simulink model "marine_otter_full"  (R2024a)
settings: Solver=FixedStepAuto  StartTime=0.0  StopTime=10.0  FixedStep=0.05  RelTol=1e-3
PostLoadFcn:
  | on_model_load
InitFcn:
  | on_model_start
StopFcn:
  | on_simulation_done
undefined symbols (not defined in the file or in its folder): ActiveExperiment
libraries: marine_lib_sys x5, data_driven_lib_ctl x3, csbenchlab_ctl x2
PostSaveFcn:
  | on_model_save
settings Model: Creator=luka  LastModifiedBy=luka

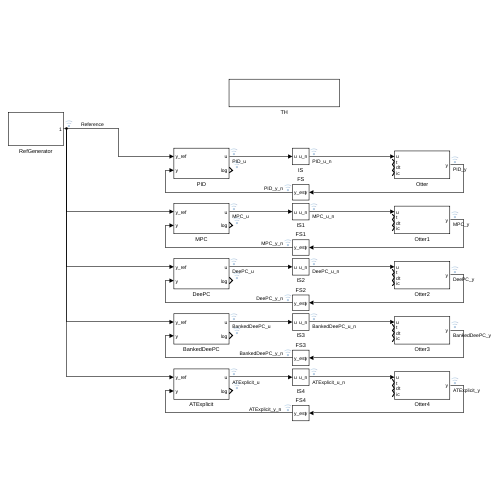
[thumbnail: Simulink's stored preview of the top-level diagram]
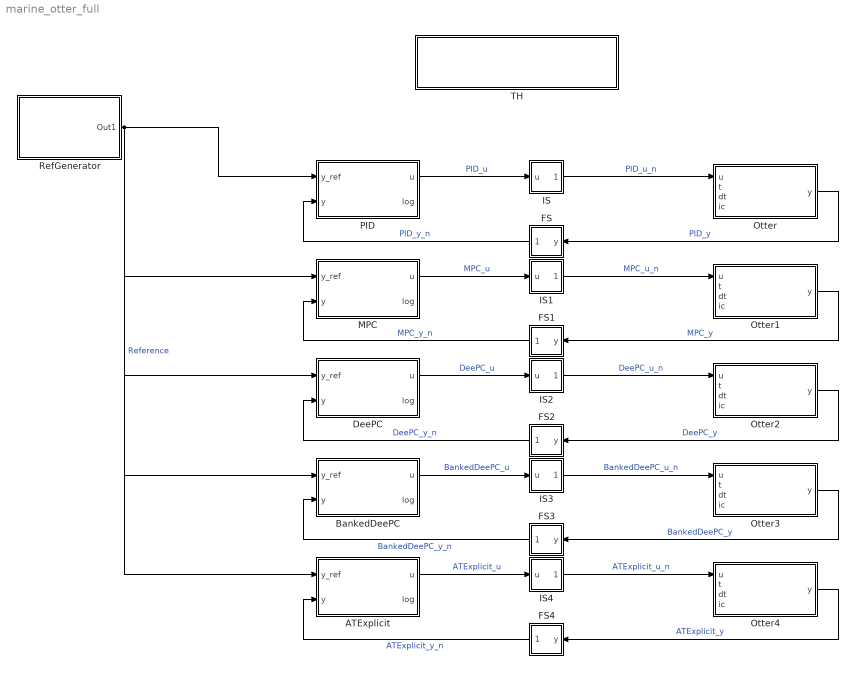
== system marine_otter_full ==
  ATExplicit : Subsystem  Tag=__cs_template;__cs_comptype:ctl
      mask DialogControl ParameterGroupVar Prompt: Params
  BankedDeePC : Subsystem  Tag=__cs_template;__cs_comptype:ctl
      mask DialogControl ParameterGroupVar Prompt: Params
  DeePC : Subsystem  Tag=__cs_template;__cs_comptype:ctl
      mask DialogControl ParameterGroupVar Prompt: Params
  FS : Subsystem
  FS1 : Subsystem
  FS2 : Subsystem
  FS3 : Subsystem
  FS4 : Subsystem
  IS : Subsystem
  IS1 : Subsystem
  IS2 : Subsystem
  IS3 : Subsystem
  IS4 : Subsystem
  MPC : Subsystem  Tag=__cs_template;__cs_comptype:ctl
      mask DialogControl ParameterGroupVar Prompt: Params
  Otter : Subsystem  Tag=__cs_template;__cs_comptype:sys
      mask DialogControl ParameterGroupVar Prompt: Params
  Otter1 : Subsystem  Tag=__cs_template;__cs_comptype:sys
      mask DialogControl ParameterGroupVar Prompt: Params
  Otter2 : Subsystem  Tag=__cs_template;__cs_comptype:sys
      mask DialogControl ParameterGroupVar Prompt: Params
  Otter3 : Subsystem  Tag=__cs_template;__cs_comptype:sys
      mask DialogControl ParameterGroupVar Prompt: Params
  Otter4 : Subsystem  Tag=__cs_template;__cs_comptype:sys
      mask DialogControl ParameterGroupVar Prompt: Params
  PID : Subsystem  Tag=__cs_template;__cs_comptype:ctl
      mask DialogControl ParameterGroupVar Prompt: Params
  RefGenerator : Subsystem  mask{experiment=P1}
      settings: OpenFcn=on_reference_generator_open();
      mask TypeOptions experiment: P1
      mask Callback experiment: on_experiment_select;
      mask DialogControl DescGroupVar Prompt: Select experiment
  TH : Subsystem
      mask DialogControl ParameterGroupVar Prompt: Params
  wires:
  PID/1(u) -> IS/1(u)  "PID_u"
  IS/1(u_n) -> Otter/1(u)  "PID_u_n"
  Otter/1(y) -> FS/1(y)  "PID_y"
  FS/1(y_est) -> PID/2(y)  "PID_y_n"
  RefGenerator/1(Out1) -> PID/1(y_ref), MPC/1(y_ref), DeePC/1(y_ref), BankedDeePC/1(y_ref), ATExplicit/1(y_ref)  "Reference"
  MPC/1(u) -> IS1/1(u)  "MPC_u"
  IS1/1(u_n) -> Otter1/1(u)  "MPC_u_n"
  Otter1/1(y) -> FS1/1(y)  "MPC_y"
  FS1/1(y_est) -> MPC/2(y)  "MPC_y_n"
  DeePC/1(u) -> IS2/1(u)  "DeePC_u"
  IS2/1(u_n) -> Otter2/1(u)  "DeePC_u_n"
  Otter2/1(y) -> FS2/1(y)  "DeePC_y"
  FS2/1(y_est) -> DeePC/2(y)  "DeePC_y_n"
  BankedDeePC/1(u) -> IS3/1(u)  "BankedDeePC_u"
  IS3/1(u_n) -> Otter3/1(u)  "BankedDeePC_u_n"
  Otter3/1(y) -> FS3/1(y)  "BankedDeePC_y"
  FS3/1(y_est) -> BankedDeePC/2(y)  "BankedDeePC_y_n"
  ATExplicit/1(u) -> IS4/1(u)  "ATExplicit_u"
  IS4/1(u_n) -> Otter4/1(u)  "ATExplicit_u_n"
  Otter4/1(y) -> FS4/1(y)  "ATExplicit_y"
  FS4/1(y_est) -> ATExplicit/2(y)  "ATExplicit_y_n"

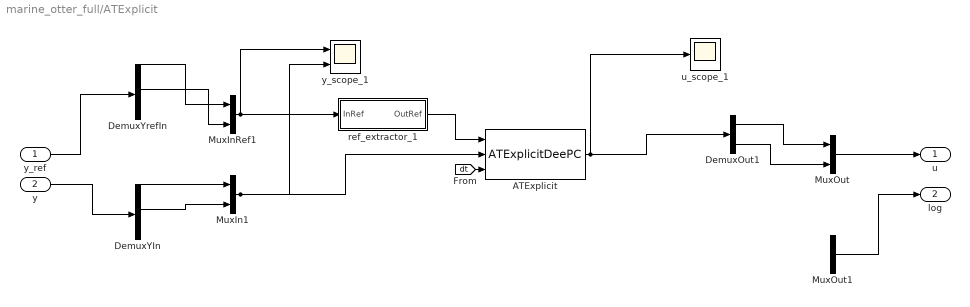
== system marine_otter_full/ATExplicit ==
  y_ref : Inport  PortDimensions=12
  y : Inport  Port=2  PortDimensions=12
  ATExplicit : data_driven_lib_ctl/ATExplicitDeePC  Tag=__cs_comptype:ctl;__cs_compimpl:mat;  iid__=[51 50 99 48 56 97 99 98 45 57 52 54 52 45 52 97 98 97 45 97 97 97 101 45 49 100 57 57 102 51 57 52 98 51 53 48]  pid__=[65 84 69 120 112 108 105 99 105 116 68 101 101 80 67 58 100 97 116 97 95 100 114 105 118 101 110 95 108 105 98]  params=marine_otter_full_params.ctl.ATExplicit  data=ATExplicitDeePC_data  ParamsType=ATExplicitDeePC_PT  DataType=ATExplicitDeePC_DT  u_ic=0
  DemuxOut1 : Demux  Outputs=2
  DemuxYIn : Demux  Outputs=12
  DemuxYrefIn : Demux  Outputs=12
  MuxIn1 : Mux  Inputs=2
  MuxInRef1 : Mux  Inputs=2
  MuxOut : Mux  Inputs=2
  MuxOut1 : BusCreator  Inputs=1
  ref_extractor_1 : Subsystem
  u_scope_1 : Scope
  y_scope_1 : Scope  NumInputPorts=2
  u : Outport  PortDimensions=2
  log : Outport  Port=2
  wires:
  [dt] -> ATExplicit/3
  y/1 -> DemuxYIn/1
  y_ref/1 -> DemuxYrefIn/1
  MuxOut/1 -> u/1
  MuxOut1/1 -> log/1
  MuxInRef1/1 -> ref_extractor_1/1(InRef), y_scope_1/1
  ref_extractor_1/1(OutRef) -> ATExplicit/1
  MuxIn1/1 -> ATExplicit/2, y_scope_1/2
  ATExplicit/1 -> DemuxOut1/1, u_scope_1/1
  DemuxYIn/1 -> MuxIn1/1
  DemuxYrefIn/1 -> MuxInRef1/1
  DemuxYIn/6 -> MuxIn1/2
  DemuxYrefIn/6 -> MuxInRef1/2
  DemuxOut1/1 -> MuxOut/1
  DemuxOut1/2 -> MuxOut/2

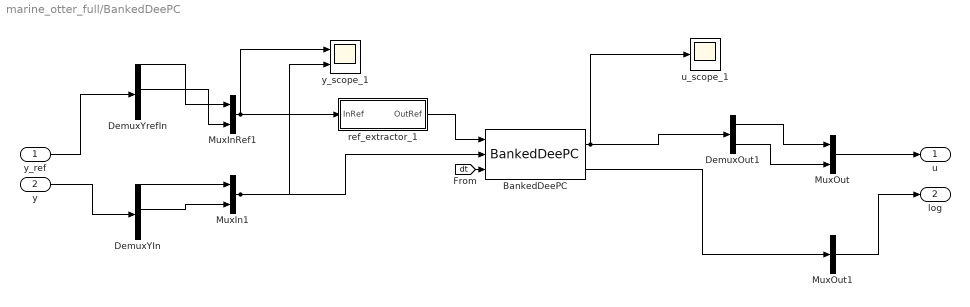
== system marine_otter_full/BankedDeePC ==
  y_ref : Inport  PortDimensions=12
  y : Inport  Port=2  PortDimensions=12
  BankedDeePC : data_driven_lib_ctl/BankedDeePC  Tag=__cs_comptype:ctl;__cs_compimpl:mat;  iid__=[54 56 49 56 55 102 55 100 45 56 49 102 53 45 52 55 53 54 45 57 54 98 101 45 100 101 48 100 54 53 51 54 51 97 54 51]  pid__=[66 97 110 107 101 100 68 101 101 80 67 58 100 97 116 97 95 100 114 105 118 101 110 95 108 105 98]  params=marine_otter_full_params.ctl.BankedDeePC  LogEntryType=BankedDeePC_LT  data=BankedDeePC_data  ParamsType=BankedDeePC_PT  DataType=BankedDeePC_DT  u_ic=0
  DemuxOut1 : Demux  Outputs=2
  DemuxYIn : Demux  Outputs=12
  DemuxYrefIn : Demux  Outputs=12
  MuxIn1 : Mux  Inputs=2
  MuxInRef1 : Mux  Inputs=2
  MuxOut : Mux  Inputs=2
  MuxOut1 : BusCreator  Inputs=1
  ref_extractor_1 : Subsystem
  u_scope_1 : Scope
  y_scope_1 : Scope  NumInputPorts=2
  u : Outport  PortDimensions=2
  log : Outport  Port=2
  wires:
  [dt] -> BankedDeePC/3
  y/1 -> DemuxYIn/1
  y_ref/1 -> DemuxYrefIn/1
  MuxOut/1 -> u/1
  MuxOut1/1 -> log/1
  MuxInRef1/1 -> ref_extractor_1/1(InRef), y_scope_1/1
  ref_extractor_1/1(OutRef) -> BankedDeePC/1
  MuxIn1/1 -> BankedDeePC/2, y_scope_1/2
  BankedDeePC/1 -> DemuxOut1/1, u_scope_1/1
  BankedDeePC/2 -> MuxOut1/1
  DemuxYIn/1 -> MuxIn1/1
  DemuxYrefIn/1 -> MuxInRef1/1
  DemuxYIn/6 -> MuxIn1/2
  DemuxYrefIn/6 -> MuxInRef1/2
  DemuxOut1/1 -> MuxOut/1
  DemuxOut1/2 -> MuxOut/2

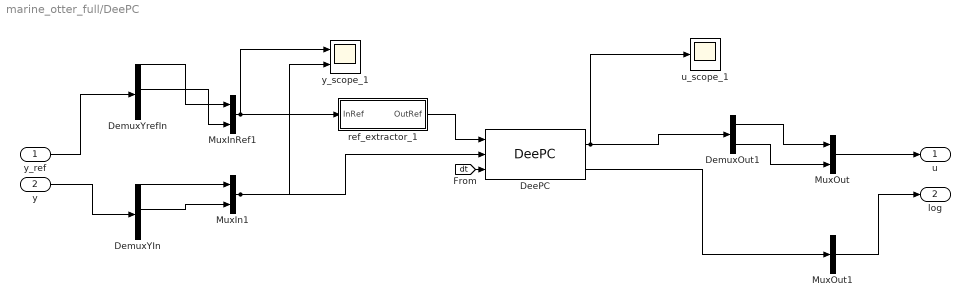
== system marine_otter_full/DeePC ==
  y_ref : Inport  PortDimensions=12
  y : Inport  Port=2  PortDimensions=12
  DeePC : data_driven_lib_ctl/DeePC  Tag=__cs_comptype:ctl;__cs_compimpl:mat;  iid__=[102 52 49 101 102 57 101 52 45 98 97 51 52 45 52 49 54 99 45 56 52 98 54 45 55 55 57 52 57 53 54 97 51 99 48 52]  pid__=[68 101 101 80 67 58 100 97 116 97 95 100 114 105 118 101 110 95 108 105 98]  params=marine_otter_full_params.ctl.DeePC  LogEntryType=DeePC_LT  data=DeePC_data  ParamsType=DeePC_PT  DataType=DeePC_DT  u_ic=0
  DemuxOut1 : Demux  Outputs=2
  DemuxYIn : Demux  Outputs=12
  DemuxYrefIn : Demux  Outputs=12
  MuxIn1 : Mux  Inputs=2
  MuxInRef1 : Mux  Inputs=2
  MuxOut : Mux  Inputs=2
  MuxOut1 : BusCreator  Inputs=1
  ref_extractor_1 : Subsystem
  u_scope_1 : Scope
  y_scope_1 : Scope  NumInputPorts=2
  u : Outport  PortDimensions=2
  log : Outport  Port=2
  wires:
  [dt] -> DeePC/3
  y/1 -> DemuxYIn/1
  y_ref/1 -> DemuxYrefIn/1
  MuxOut/1 -> u/1
  MuxOut1/1 -> log/1
  MuxInRef1/1 -> ref_extractor_1/1(InRef), y_scope_1/1
  ref_extractor_1/1(OutRef) -> DeePC/1
  MuxIn1/1 -> DeePC/2, y_scope_1/2
  DeePC/1 -> DemuxOut1/1, u_scope_1/1
  DeePC/2 -> MuxOut1/1
  DemuxYIn/1 -> MuxIn1/1
  DemuxYrefIn/1 -> MuxInRef1/1
  DemuxYIn/6 -> MuxIn1/2
  DemuxYrefIn/6 -> MuxInRef1/2
  DemuxOut1/1 -> MuxOut/1
  DemuxOut1/2 -> MuxOut/2

== system marine_otter_full/FS ==
  y : Inport
  CS Dist : Subsystem
      mask DialogControl ParameterGroupVar Prompt: Params
  CS Est : Subsystem
      mask DialogControl ParameterGroupVar Prompt: Params
  y_est : Outport
  wires:
  CS Est/1(y_est) -> y_est/1
  CS Dist/1(y_n) -> CS Est/1(y)
  y/1 -> CS Dist/1(y)

== system marine_otter_full/FS1 ==
  y : Inport
  CS Dist : Subsystem
      mask DialogControl ParameterGroupVar Prompt: Params
  CS Est : Subsystem
      mask DialogControl ParameterGroupVar Prompt: Params
  y_est : Outport
  wires:
  CS Est/1(y_est) -> y_est/1
  CS Dist/1(y_n) -> CS Est/1(y)
  y/1 -> CS Dist/1(y)

== system marine_otter_full/FS2 ==
  y : Inport
  CS Dist : Subsystem
      mask DialogControl ParameterGroupVar Prompt: Params
  CS Est : Subsystem
      mask DialogControl ParameterGroupVar Prompt: Params
  y_est : Outport
  wires:
  CS Est/1(y_est) -> y_est/1
  CS Dist/1(y_n) -> CS Est/1(y)
  y/1 -> CS Dist/1(y)

== system marine_otter_full/FS3 ==
  y : Inport
  CS Dist : Subsystem
      mask DialogControl ParameterGroupVar Prompt: Params
  CS Est : Subsystem
      mask DialogControl ParameterGroupVar Prompt: Params
  y_est : Outport
  wires:
  CS Est/1(y_est) -> y_est/1
  CS Dist/1(y_n) -> CS Est/1(y)
  y/1 -> CS Dist/1(y)

== system marine_otter_full/FS4 ==
  y : Inport
  CS Dist : Subsystem
      mask DialogControl ParameterGroupVar Prompt: Params
  CS Est : Subsystem
      mask DialogControl ParameterGroupVar Prompt: Params
  y_est : Outport
  wires:
  CS Est/1(y_est) -> y_est/1
  CS Dist/1(y_n) -> CS Est/1(y)
  y/1 -> CS Dist/1(y)

== system marine_otter_full/IS ==
  u : Inport
  CS Dist : Subsystem
      mask DialogControl ParameterGroupVar Prompt: Params
  u_n : Outport
  wires:
  CS Dist/1(y_n) -> u_n/1
  u/1 -> CS Dist/1(y)

== system marine_otter_full/IS1 ==
  u : Inport
  CS Dist : Subsystem
      mask DialogControl ParameterGroupVar Prompt: Params
  u_n : Outport
  wires:
  CS Dist/1(y_n) -> u_n/1
  u/1 -> CS Dist/1(y)

== system marine_otter_full/IS2 ==
  u : Inport
  CS Dist : Subsystem
      mask DialogControl ParameterGroupVar Prompt: Params
  u_n : Outport
  wires:
  CS Dist/1(y_n) -> u_n/1
  u/1 -> CS Dist/1(y)

== system marine_otter_full/IS3 ==
  u : Inport
  CS Dist : Subsystem
      mask DialogControl ParameterGroupVar Prompt: Params
  u_n : Outport
  wires:
  CS Dist/1(y_n) -> u_n/1
  u/1 -> CS Dist/1(y)

== system marine_otter_full/IS4 ==
  u : Inport
  CS Dist : Subsystem
      mask DialogControl ParameterGroupVar Prompt: Params
  u_n : Outport
  wires:
  CS Dist/1(y_n) -> u_n/1
  u/1 -> CS Dist/1(y)

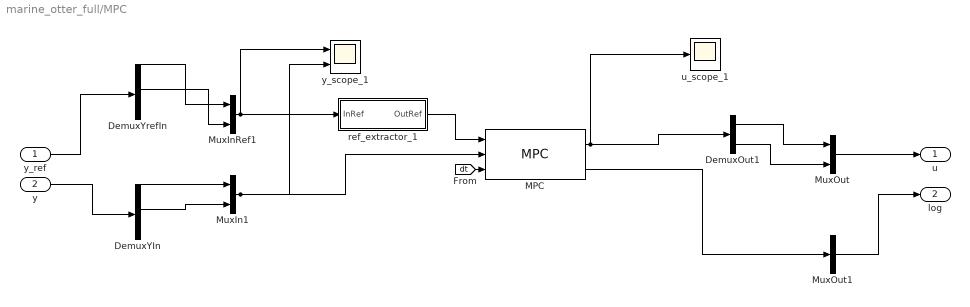
== system marine_otter_full/MPC ==
  y_ref : Inport  PortDimensions=12
  y : Inport  Port=2  PortDimensions=12
  DemuxOut1 : Demux  Outputs=2
  DemuxYIn : Demux  Outputs=12
  DemuxYrefIn : Demux  Outputs=12
  MPC : csbenchlab_ctl/MPC  Tag=__cs_slx_ctl;__cs_comptype:ctl;__cs_compimpl:slx;  mpc_path=0  out_gain=0  iid__=[56 49 102 99 48 101 54 102 45 50 51 56 52 45 52 57 54 57 45 97 98 51 51 45 52 99 99 48 98 52 97 56 56 100 97 99]  pid__=[77 80 67 58 99 115 98 101 110 99 104 108 97 98]  params=marine_otter_full_params.ctl.MPC  params_struct_name=marine_otter_full_params.ctl.MPC
  MuxIn1 : Mux  Inputs=2
  MuxInRef1 : Mux  Inputs=2
  MuxOut : Mux  Inputs=2
  MuxOut1 : BusCreator  Inputs=1
  ref_extractor_1 : Subsystem
  u_scope_1 : Scope
  y_scope_1 : Scope  NumInputPorts=2
  u : Outport  PortDimensions=2
  log : Outport  Port=2
  wires:
  [dt] -> MPC/3
  y/1 -> DemuxYIn/1
  y_ref/1 -> DemuxYrefIn/1
  MuxOut/1 -> u/1
  MuxOut1/1 -> log/1
  MuxInRef1/1 -> ref_extractor_1/1(InRef), y_scope_1/1
  ref_extractor_1/1(OutRef) -> MPC/1
  MuxIn1/1 -> MPC/2, y_scope_1/2
  MPC/1 -> DemuxOut1/1, u_scope_1/1
  MPC/2 -> MuxOut1/1
  DemuxYIn/1 -> MuxIn1/1
  DemuxYrefIn/1 -> MuxInRef1/1
  DemuxYIn/6 -> MuxIn1/2
  DemuxYrefIn/6 -> MuxInRef1/2
  DemuxOut1/1 -> MuxOut/1
  DemuxOut1/2 -> MuxOut/2

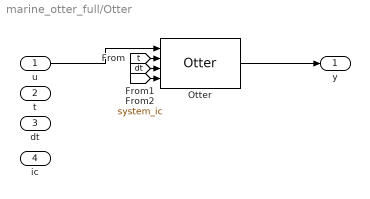
== system marine_otter_full/Otter ==
  u : Inport
  t : Inport  Port=2
  dt : Inport  Port=3
  ic : Inport  Port=4
  Otter : marine_lib_sys/Otter  Tag=system;__cs_slx_sys;__cs_comptype:sys;__cs_compimpl:slx;  payload_mass=0  payload_location=[0,0, 0]  current_speed=0  current_direction=0  out_gain=1  iid__=[52 97 48 100 49 48 49 48 45 52 53 52 57 45 52 100 53 49 45 98 51 97 53 45 54 48 50 101 55 99 57 51 50 98 52 53]  pid__=[79 116 116 101 114 58 109 97 114 105 110 101 95 108 105 98]  params=ActiveExperiment.SystemParams  params_struct_name=marine_otter_full_params.sys.Otter
  y : Outport
  wires:
  u/1 -> Otter/1
  Otter/1 -> y/1
  [t] -> Otter/2
  [dt] -> Otter/3
  [system_ic] -> Otter/4

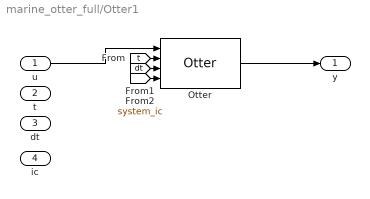
== system marine_otter_full/Otter1 ==
  u : Inport
  t : Inport  Port=2
  dt : Inport  Port=3
  ic : Inport  Port=4
  Otter : marine_lib_sys/Otter  Tag=system;__cs_slx_sys;__cs_comptype:sys;__cs_compimpl:slx;  payload_mass=0  payload_location=[0,0, 0]  current_speed=0  current_direction=0  out_gain=1  iid__=[52 97 48 100 49 48 49 48 45 52 53 52 57 45 52 100 53 49 45 98 51 97 53 45 54 48 50 101 55 99 57 51 50 98 52 53]  pid__=[79 116 116 101 114 58 109 97 114 105 110 101 95 108 105 98]  params=ActiveExperiment.SystemParams  params_struct_name=marine_otter_full_params.sys.Otter
  y : Outport
  wires:
  u/1 -> Otter/1
  Otter/1 -> y/1
  [t] -> Otter/2
  [dt] -> Otter/3
  [system_ic] -> Otter/4

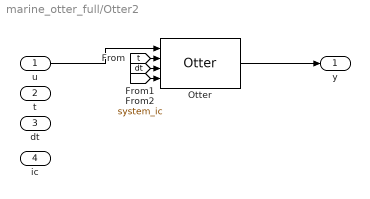
== system marine_otter_full/Otter2 ==
  u : Inport
  t : Inport  Port=2
  dt : Inport  Port=3
  ic : Inport  Port=4
  Otter : marine_lib_sys/Otter  Tag=system;__cs_slx_sys;__cs_comptype:sys;__cs_compimpl:slx;  payload_mass=0  payload_location=[0,0, 0]  current_speed=0  current_direction=0  out_gain=1  iid__=[52 97 48 100 49 48 49 48 45 52 53 52 57 45 52 100 53 49 45 98 51 97 53 45 54 48 50 101 55 99 57 51 50 98 52 53]  pid__=[79 116 116 101 114 58 109 97 114 105 110 101 95 108 105 98]  params=ActiveExperiment.SystemParams  params_struct_name=marine_otter_full_params.sys.Otter
  y : Outport
  wires:
  u/1 -> Otter/1
  Otter/1 -> y/1
  [t] -> Otter/2
  [dt] -> Otter/3
  [system_ic] -> Otter/4

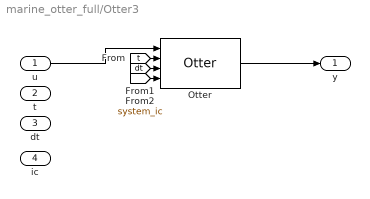
== system marine_otter_full/Otter3 ==
  u : Inport
  t : Inport  Port=2
  dt : Inport  Port=3
  ic : Inport  Port=4
  Otter : marine_lib_sys/Otter  Tag=system;__cs_slx_sys;__cs_comptype:sys;__cs_compimpl:slx;  payload_mass=0  payload_location=[0,0, 0]  current_speed=0  current_direction=0  out_gain=1  iid__=[52 97 48 100 49 48 49 48 45 52 53 52 57 45 52 100 53 49 45 98 51 97 53 45 54 48 50 101 55 99 57 51 50 98 52 53]  pid__=[79 116 116 101 114 58 109 97 114 105 110 101 95 108 105 98]  params=ActiveExperiment.SystemParams  params_struct_name=marine_otter_full_params.sys.Otter
  y : Outport
  wires:
  u/1 -> Otter/1
  Otter/1 -> y/1
  [t] -> Otter/2
  [dt] -> Otter/3
  [system_ic] -> Otter/4

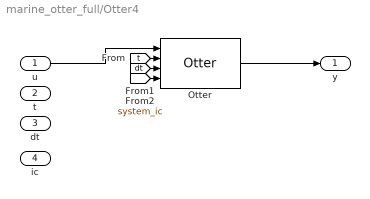
== system marine_otter_full/Otter4 ==
  u : Inport
  t : Inport  Port=2
  dt : Inport  Port=3
  ic : Inport  Port=4
  Otter : marine_lib_sys/Otter  Tag=system;__cs_slx_sys;__cs_comptype:sys;__cs_compimpl:slx;  payload_mass=0  payload_location=[0,0, 0]  current_speed=0  current_direction=0  out_gain=1  iid__=[52 97 48 100 49 48 49 48 45 52 53 52 57 45 52 100 53 49 45 98 51 97 53 45 54 48 50 101 55 99 57 51 50 98 52 53]  pid__=[79 116 116 101 114 58 109 97 114 105 110 101 95 108 105 98]  params=ActiveExperiment.SystemParams  params_struct_name=marine_otter_full_params.sys.Otter
  y : Outport
  wires:
  u/1 -> Otter/1
  Otter/1 -> y/1
  [t] -> Otter/2
  [dt] -> Otter/3
  [system_ic] -> Otter/4

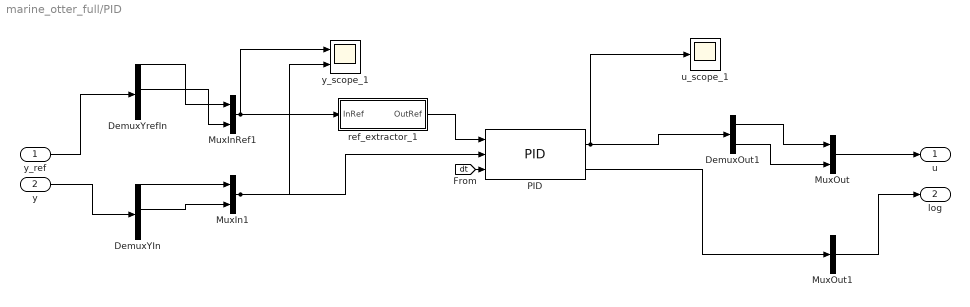
== system marine_otter_full/PID ==
  y_ref : Inport  PortDimensions=12
  y : Inport  Port=2  PortDimensions=12
  DemuxOut1 : Demux  Outputs=2
  DemuxYIn : Demux  Outputs=12
  DemuxYrefIn : Demux  Outputs=12
  MuxIn1 : Mux  Inputs=2
  MuxInRef1 : Mux  Inputs=2
  MuxOut : Mux  Inputs=2
  MuxOut1 : BusCreator  Inputs=1
  PID : csbenchlab_ctl/PID  Tag=__cs_slx_ctl;__cs_comptype:ctl;__cs_compimpl:slx;  K_p=K_p  K_i=K_i  K_d=K_d  K_N=K_N  saturation_min=saturation_min  saturation_max=saturation_max  iid__=[56 53 56 50 101 51 101 49 45 100 101 56 53 45 52 54 54 101 45 98 52 49 50 45 52 52 97 50 54 57 99 99 100 50 98 102]  pid__=[80 73 68 58 99 115 98 101 110 99 104 108 97 98]  params=marine_otter_full_params.ctl.PID  params_struct_name=marine_otter_full_params.ctl.PID
  ref_extractor_1 : Subsystem
  u_scope_1 : Scope
  y_scope_1 : Scope  NumInputPorts=2
  u : Outport  PortDimensions=2
  log : Outport  Port=2
  wires:
  [dt] -> PID/3
  y/1 -> DemuxYIn/1
  y_ref/1 -> DemuxYrefIn/1
  MuxOut/1 -> u/1
  MuxOut1/1 -> log/1
  MuxInRef1/1 -> ref_extractor_1/1(InRef), y_scope_1/1
  ref_extractor_1/1(OutRef) -> PID/1
  MuxIn1/1 -> PID/2, y_scope_1/2
  PID/1 -> DemuxOut1/1, u_scope_1/1
  PID/2 -> MuxOut1/1
  DemuxYIn/1 -> MuxIn1/1
  DemuxYrefIn/1 -> MuxInRef1/1
  DemuxYIn/6 -> MuxIn1/2
  DemuxYrefIn/6 -> MuxInRef1/2
  DemuxOut1/1 -> MuxOut/1
  DemuxOut1/2 -> MuxOut/2

== system marine_otter_full/RefGenerator ==
  IC : Constant  Value=ActiveExperiment.SystemIc
  ReferenceFile : FromFile  SampleTime=0
  Out1 : Outport
  tag scope: system_ic=global
  wires:
  IC/1 -> [system_ic]
  ReferenceFile/1 -> Out1/1

== system marine_otter_full/TH ==
  Clock : Clock
  Constant : Constant
  Memory : Memory
  Subtract : Sum  Inputs=+-
  tag scope: dt=global, t=global
  wires:
  Subtract/1 -> [dt]
  Memory/1 -> Subtract/2
  Clock/1 -> Memory/1, Subtract/1, [t]

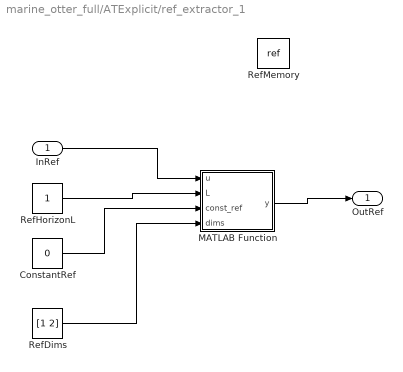
== system marine_otter_full/ATExplicit/ref_extractor_1 ==
  InRef : Inport
  ConstantRef : Constant  Value=0
  MATLAB Function : MATLAB Function  TreatAsAtomicUnit=on
  RefDims : Constant  Value=[1 2]
  RefHorizonL : Constant
  RefMemory : DataStoreMemory  DataStoreName=ref  WriteAfterWriteMsg=warning  ShowAdditionalParam=off  OutDataTypeStr=double
  OutRef : Outport
  wires:
  ConstantRef/1 -> MATLAB Function/3(const_ref)
  RefDims/1 -> MATLAB Function/4(dims)
  RefHorizonL/1 -> MATLAB Function/2(L)
  InRef/1 -> MATLAB Function/1(u)
  MATLAB Function/1(y) -> OutRef/1

== system marine_otter_full/BankedDeePC/ref_extractor_1 ==
  InRef : Inport
  ConstantRef : Constant  Value=0
  MATLAB Function : MATLAB Function  TreatAsAtomicUnit=on
  RefDims : Constant  Value=[1 2]
  RefHorizonL : Constant
  RefMemory : DataStoreMemory  DataStoreName=ref  WriteAfterWriteMsg=warning  ShowAdditionalParam=off  OutDataTypeStr=double
  OutRef : Outport
  wires:
  ConstantRef/1 -> MATLAB Function/3(const_ref)
  RefDims/1 -> MATLAB Function/4(dims)
  RefHorizonL/1 -> MATLAB Function/2(L)
  InRef/1 -> MATLAB Function/1(u)
  MATLAB Function/1(y) -> OutRef/1

== system marine_otter_full/DeePC/ref_extractor_1 ==
  InRef : Inport
  ConstantRef : Constant  Value=0
  MATLAB Function : MATLAB Function  TreatAsAtomicUnit=on
  RefDims : Constant  Value=[1 2]
  RefHorizonL : Constant
  RefMemory : DataStoreMemory  DataStoreName=ref  WriteAfterWriteMsg=warning  ShowAdditionalParam=off  OutDataTypeStr=double
  OutRef : Outport
  wires:
  ConstantRef/1 -> MATLAB Function/3(const_ref)
  RefDims/1 -> MATLAB Function/4(dims)
  RefHorizonL/1 -> MATLAB Function/2(L)
  InRef/1 -> MATLAB Function/1(u)
  MATLAB Function/1(y) -> OutRef/1

== system marine_otter_full/FS/CS Dist ==
  y : Inport
  Gain : Gain
  y_n : Outport
  wires:
  Gain/1 -> y_n/1
  y/1 -> Gain/1

== system marine_otter_full/FS/CS Est ==
  y : Inport
  Gain : Gain
  y_est : Outport
  wires:
  y/1 -> Gain/1
  Gain/1 -> y_est/1

== system marine_otter_full/FS1/CS Dist ==
  y : Inport
  Gain : Gain
  y_n : Outport
  wires:
  Gain/1 -> y_n/1
  y/1 -> Gain/1

== system marine_otter_full/FS1/CS Est ==
  y : Inport
  Gain : Gain
  y_est : Outport
  wires:
  y/1 -> Gain/1
  Gain/1 -> y_est/1

== system marine_otter_full/FS2/CS Dist ==
  y : Inport
  Gain : Gain
  y_n : Outport
  wires:
  Gain/1 -> y_n/1
  y/1 -> Gain/1

== system marine_otter_full/FS2/CS Est ==
  y : Inport
  Gain : Gain
  y_est : Outport
  wires:
  y/1 -> Gain/1
  Gain/1 -> y_est/1

== system marine_otter_full/FS3/CS Dist ==
  y : Inport
  Gain : Gain
  y_n : Outport
  wires:
  Gain/1 -> y_n/1
  y/1 -> Gain/1

== system marine_otter_full/FS3/CS Est ==
  y : Inport
  Gain : Gain
  y_est : Outport
  wires:
  y/1 -> Gain/1
  Gain/1 -> y_est/1

== system marine_otter_full/FS4/CS Dist ==
  y : Inport
  Gain : Gain
  y_n : Outport
  wires:
  Gain/1 -> y_n/1
  y/1 -> Gain/1

== system marine_otter_full/FS4/CS Est ==
  y : Inport
  Gain : Gain
  y_est : Outport
  wires:
  y/1 -> Gain/1
  Gain/1 -> y_est/1

== system marine_otter_full/IS/CS Dist ==
  y : Inport
  Gain : Gain
  y_n : Outport
  wires:
  y/1 -> Gain/1
  Gain/1 -> y_n/1

== system marine_otter_full/IS1/CS Dist ==
  y : Inport
  Gain : Gain
  y_n : Outport
  wires:
  y/1 -> Gain/1
  Gain/1 -> y_n/1

== system marine_otter_full/IS2/CS Dist ==
  y : Inport
  Gain : Gain
  y_n : Outport
  wires:
  y/1 -> Gain/1
  Gain/1 -> y_n/1

== system marine_otter_full/IS3/CS Dist ==
  y : Inport
  Gain : Gain
  y_n : Outport
  wires:
  y/1 -> Gain/1
  Gain/1 -> y_n/1

== system marine_otter_full/IS4/CS Dist ==
  y : Inport
  Gain : Gain
  y_n : Outport
  wires:
  y/1 -> Gain/1
  Gain/1 -> y_n/1

== system marine_otter_full/MPC/ref_extractor_1 ==
  InRef : Inport
  ConstantRef : Constant  Value=0
  MATLAB Function : MATLAB Function  TreatAsAtomicUnit=on
  RefDims : Constant  Value=[1 2]
  RefHorizonL : Constant
  RefMemory : DataStoreMemory  DataStoreName=ref  WriteAfterWriteMsg=warning  ShowAdditionalParam=off  OutDataTypeStr=double
  OutRef : Outport
  wires:
  ConstantRef/1 -> MATLAB Function/3(const_ref)
  RefDims/1 -> MATLAB Function/4(dims)
  RefHorizonL/1 -> MATLAB Function/2(L)
  InRef/1 -> MATLAB Function/1(u)
  MATLAB Function/1(y) -> OutRef/1

== system marine_otter_full/PID/ref_extractor_1 ==
  InRef : Inport
  ConstantRef : Constant  Value=0
  MATLAB Function : MATLAB Function  TreatAsAtomicUnit=on
  RefDims : Constant  Value=[1 2]
  RefHorizonL : Constant
  RefMemory : DataStoreMemory  DataStoreName=ref  WriteAfterWriteMsg=warning  ShowAdditionalParam=off  OutDataTypeStr=double
  OutRef : Outport
  wires:
  ConstantRef/1 -> MATLAB Function/3(const_ref)
  RefDims/1 -> MATLAB Function/4(dims)
  RefHorizonL/1 -> MATLAB Function/2(L)
  InRef/1 -> MATLAB Function/1(u)
  MATLAB Function/1(y) -> OutRef/1

== matlab function marine_otter_full/MPC/ref_extractor_1/MATLAB Function ==
  settings: updateMethod=DISCRETE
  data: u input; L input; const_ref input; dims input; y output; ref data_store_memory; GlobalReference parameter
function y = fcn(u, L, const_ref, dims, GlobalReference)

persistent cnt
global ref

if isempty(cnt)
    cnt = 0;
end

if GlobalReference == 0
    y = repmat(u', 1);
    return;
end


cnt = cnt+1;

horizon_end = cnt+L-1;
if L > 1 
   if horizon_end > length(GlobalReference)
        if size(ref, 1) == size(u, 1)
            y = permute(ref, [2, 1]);
        else
            y = ref;
        end       
        return
   end

   if size(ref, 1) == size(u, 1)
      
      if const_ref == 0
        ref(:, :) = GlobalReference(cnt:horizon_end, dims)';
      else
        ref(:, :) = repmat(GlobalReference(cnt, dims)', 1, L);
      end
      y = permute(ref, [2, 1]);
   else
      if const_ref == 0
        ref(1:L, :) = GlobalReference(cnt:horizon_end, dims);
      else
        ref(1:L, :) = repmat(GlobalReference(cnt, dims), L, 1);
      end
      y = ref;
   end
else
   if size(ref, 1) == size(u, 1)
       ref = u;
       y = permute(ref, [2, 1]);
   else
      ref(1, :) = u';
      y = ref;
   end
end

== matlab function marine_otter_full/DeePC/ref_extractor_1/MATLAB Function ==
  settings: updateMethod=DISCRETE
  data: u input; L input; const_ref input; dims input; y output; ref data_store_memory; GlobalReference parameter
function y = fcn(u, L, const_ref, dims, GlobalReference)

persistent cnt
global ref

if isempty(cnt)
    cnt = 0;
end

if GlobalReference == 0
    y = repmat(u', 1);
    return;
end


cnt = cnt+1;

horizon_end = cnt+L-1;
if L > 1 
   if horizon_end > length(GlobalReference)
        if size(ref, 1) == size(u, 1)
            y = permute(ref, [2, 1]);
        else
            y = ref;
        end       
        return
   end

   if size(ref, 1) == size(u, 1)
      
      if const_ref == 0
        ref(:, :) = GlobalReference(cnt:horizon_end, dims)';
      else
        ref(:, :) = repmat(GlobalReference(cnt, dims)', 1, L);
      end
      y = permute(ref, [2, 1]);
   else
      if const_ref == 0
        ref(1:L, :) = GlobalReference(cnt:horizon_end, dims);
      else
        ref(1:L, :) = repmat(GlobalReference(cnt, dims), L, 1);
      end
      y = ref;
   end
else
   if size(ref, 1) == size(u, 1)
       ref = u;
       y = permute(ref, [2, 1]);
   else
      ref(1, :) = u';
      y = ref;
   end
end

== matlab function marine_otter_full/BankedDeePC/ref_extractor_1/MATLAB Function ==
  settings: updateMethod=DISCRETE
  data: u input; L input; const_ref input; dims input; y output; ref data_store_memory; GlobalReference parameter
function y = fcn(u, L, const_ref, dims, GlobalReference)

persistent cnt
global ref

if isempty(cnt)
    cnt = 0;
end

if GlobalReference == 0
    y = repmat(u', 1);
    return;
end


cnt = cnt+1;

horizon_end = cnt+L-1;
if L > 1 
   if horizon_end > length(GlobalReference)
        if size(ref, 1) == size(u, 1)
            y = permute(ref, [2, 1]);
        else
            y = ref;
        end       
        return
   end

   if size(ref, 1) == size(u, 1)
      
      if const_ref == 0
        ref(:, :) = GlobalReference(cnt:horizon_end, dims)';
      else
        ref(:, :) = repmat(GlobalReference(cnt, dims)', 1, L);
      end
      y = permute(ref, [2, 1]);
   else
      if const_ref == 0
        ref(1:L, :) = GlobalReference(cnt:horizon_end, dims);
      else
        ref(1:L, :) = repmat(GlobalReference(cnt, dims), L, 1);
      end
      y = ref;
   end
else
   if size(ref, 1) == size(u, 1)
       ref = u;
       y = permute(ref, [2, 1]);
   else
      ref(1, :) = u';
      y = ref;
   end
end

== matlab function marine_otter_full/ATExplicit/ref_extractor_1/MATLAB Function ==
  settings: updateMethod=DISCRETE
  data: u input; L input; const_ref input; dims input; y output; ref data_store_memory; GlobalReference parameter
function y = fcn(u, L, const_ref, dims, GlobalReference)

persistent cnt
global ref

if isempty(cnt)
    cnt = 0;
end

if GlobalReference == 0
    y = repmat(u', 1);
    return;
end


cnt = cnt+1;

horizon_end = cnt+L-1;
if L > 1 
   if horizon_end > length(GlobalReference)
        if size(ref, 1) == size(u, 1)
            y = permute(ref, [2, 1]);
        else
            y = ref;
        end       
        return
   end

   if size(ref, 1) == size(u, 1)
      
      if const_ref == 0
        ref(:, :) = GlobalReference(cnt:horizon_end, dims)';
      else
        ref(:, :) = repmat(GlobalReference(cnt, dims)', 1, L);
      end
      y = permute(ref, [2, 1]);
   else
      if const_ref == 0
        ref(1:L, :) = GlobalReference(cnt:horizon_end, dims);
      else
        ref(1:L, :) = repmat(GlobalReference(cnt, dims), L, 1);
      end
      y = ref;
   end
else
   if size(ref, 1) == size(u, 1)
       ref = u;
       y = permute(ref, [2, 1]);
   else
      ref(1, :) = u';
      y = ref;
   end
end

== matlab function marine_otter_full/PID/ref_extractor_1/MATLAB Function ==
  settings: updateMethod=DISCRETE
  data: u input; L input; const_ref input; dims input; y output; ref data_store_memory; GlobalReference parameter
function y = fcn(u, L, const_ref, dims, GlobalReference)

persistent cnt
global ref

if isempty(cnt)
    cnt = 0;
end

if GlobalReference == 0
    y = repmat(u', 1);
    return;
end


cnt = cnt+1;

horizon_end = cnt+L-1;
if L > 1 
   if horizon_end > length(GlobalReference)
        if size(ref, 1) == size(u, 1)
            y = permute(ref, [2, 1]);
        else
            y = ref;
        end       
        return
   end

   if size(ref, 1) == size(u, 1)
      
      if const_ref == 0
        ref(:, :) = GlobalReference(cnt:horizon_end, dims)';
      else
        ref(:, :) = repmat(GlobalReference(cnt, dims)', 1, L);
      end
      y = permute(ref, [2, 1]);
   else
      if const_ref == 0
        ref(1:L, :) = GlobalReference(cnt:horizon_end, dims);
      else
        ref(1:L, :) = repmat(GlobalReference(cnt, dims), L, 1);
      end
      y = ref;
   end
else
   if size(ref, 1) == size(u, 1)
       ref = u;
       y = permute(ref, [2, 1]);
   else
      ref(1, :) = u';
      y = ref;
   end
end
